simulink model "Sphere_Complex_Model"  (R2023a)
settings: Solver=VariableStepAuto  StartTime=0.0  StopTime=100  FixedStep=impulse_time  RelTol=1e-3
values from neighbouring files (symbols this model uses):
  Ex_Force = Command_Force(Input_F, F_Coord)    [init.m]    (also in nongrad_opt.m; obj_func.m; obj_func_plot.m)
  impulse_time = 0.001    [init.m]    (also in nongrad_opt.m; obj_func.m; obj_func_plot.m)
  Param = Sphere_Parameters(percent_foam, percent_metal)    [init.m]    (also in nongrad_opt.m = Sphere_Parameters(percent_foam(row), percent_metal(column)); obj_func.m; obj_func_plot.m = Sphere_Parameters(pf(row, column), pm(row, column)))
undefined symbols (not defined in the file or in its folder): Sphere_Model
settings Model: Creator=goks  LastModifiedBy=goks

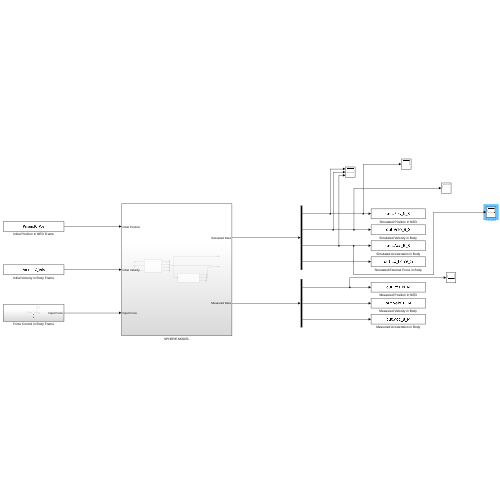
[thumbnail: Simulink's stored preview of the top-level diagram]
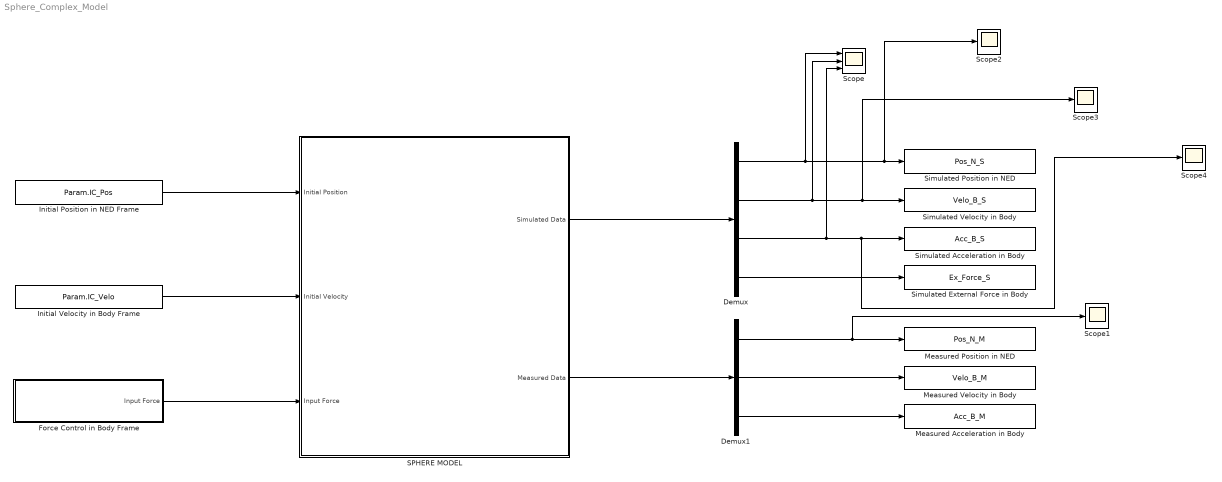
== system Sphere_Complex_Model ==
  Demux : Demux
  Demux1 : Demux  Outputs=3
  Force Control in Body Frame : Subsystem
  Initial Position in NED Frame : Constant  Value=Param.IC_Pos
  Initial Velocity in Body Frame : Constant  Value=Param.IC_Velo
  Measured Acceleration in Body : ToWorkspace  VariableName=Acc_B_M  SaveFormat=Timeseries  SampleTime=-1
  Measured Position in NED : ToWorkspace  VariableName=Pos_N_M  SaveFormat=Timeseries  SampleTime=-1
  Measured Velocity in Body : ToWorkspace  VariableName=Velo_B_M  SaveFormat=Timeseries  SampleTime=-1
  SPHERE MODEL : Subsystem
  Scope : Scope  NumInputPorts=3
  Scope{1..4} (4 alike) : Scope
  Simulated Acceleration in Body : ToWorkspace  VariableName=Acc_B_S  SaveFormat=Timeseries  SampleTime=-1
  Simulated External Force in Body : ToWorkspace  VariableName=Ex_Force_S  SaveFormat=Timeseries  SampleTime=-1
  Simulated Position in NED : ToWorkspace  VariableName=Pos_N_S  SaveFormat=Timeseries  SampleTime=-1
  Simulated Velocity in Body : ToWorkspace  VariableName=Velo_B_S  SaveFormat=Timeseries  SampleTime=-1
  wires:
  SPHERE MODEL/1(Simulated Data) -> Demux/1
  SPHERE MODEL/2(Measured Data) -> Demux1/1
  Demux/1 -> Scope/1, Scope2/1, Simulated Position in NED/1
  Demux/2 -> Scope/2, Scope3/1, Simulated Velocity in Body/1
  Demux/3 -> Scope/3, Scope4/1, Simulated Acceleration in Body/1
  Demux/4 -> Simulated External Force in Body/1
  Demux1/2 -> Measured Velocity in Body/1
  Demux1/3 -> Measured Acceleration in Body/1
  Initial Position in NED Frame/1 -> SPHERE MODEL/1("Initial Position ")
  Initial Velocity in Body Frame/1 -> SPHERE MODEL/2(Initial Velocity)
  Force Control in Body Frame/1(Input Force) -> SPHERE MODEL/3(Input Force)
  Demux1/1 -> Scope1/1, Measured Position in NED/1

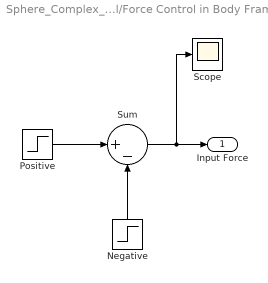
== system Sphere_Complex_Model/Force Control in Body Frame ==
  Negative : Step  Time=1+impulse_time  Before=zeros(6,1)  After=Ex_Force  SampleTime=0
  Positive : Step  Before=zeros(6,1)  After=Ex_Force  SampleTime=0
  Scope : Scope
  Sum : Sum  Inputs=|+-
  Input Force : Outport
  wires:
  Positive/1 -> Sum/1
  Negative/1 -> Sum/2
  Sum/1 -> Scope/1, Input Force/1

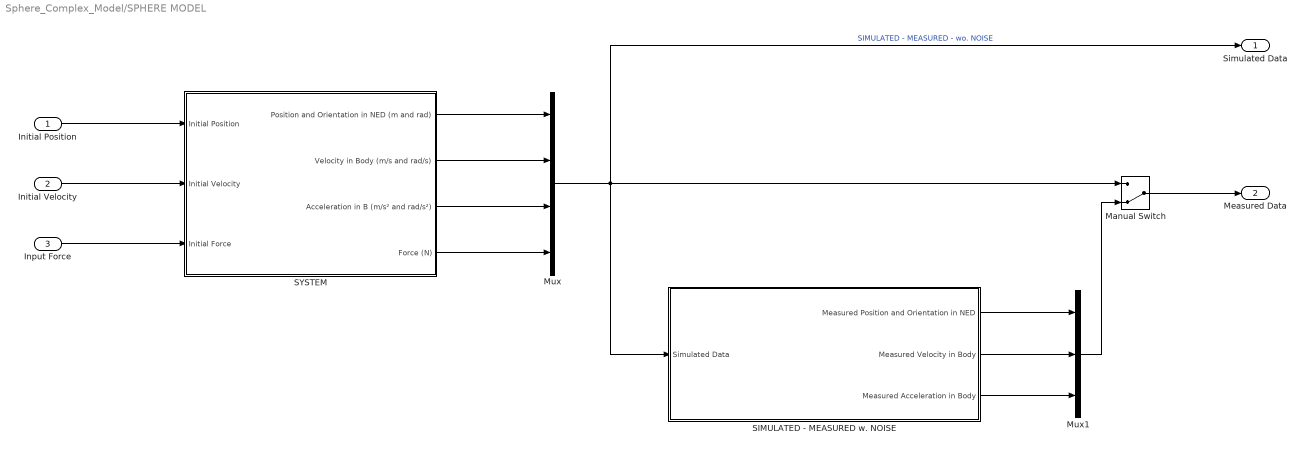
== system Sphere_Complex_Model/SPHERE MODEL ==
  "Initial Position " : Inport
  Initial Velocity : Inport  Port=2
  Input Force : Inport  Port=3
  Manual Switch : ManualSwitch  CurrentSetting=0
  Mux : Mux
  Mux1 : Mux  Inputs=3
  SIMULATED - MEASURED w. NOISE : Subsystem
  SYSTEM : Subsystem
  Simulated Data : Outport
  Measured Data : Outport  Port=2
  wires:
  SYSTEM/1(Position and Orientation in NED (m and rad)) -> Mux/1
  SYSTEM/2(Velocity in Body (m/s and rad/s)) -> Mux/2
  SYSTEM/3(Acceleration in B (m/s² and rad/s²)) -> Mux/3
  SYSTEM/4(Force (N)) -> Mux/4
  "Initial Position "/1 -> SYSTEM/1("Initial Position ")
  Initial Velocity/1 -> SYSTEM/2(Initial Velocity)
  Input Force/1 -> SYSTEM/3(Initial Force)
  SIMULATED - MEASURED w. NOISE/2(Measured Velocity in Body) -> Mux1/2
  SIMULATED - MEASURED w. NOISE/1(Measured Position and Orientation in NED) -> Mux1/1
  SIMULATED - MEASURED w. NOISE/3(Measured Acceleration in Body) -> Mux1/3
  Mux/1 -> SIMULATED - MEASURED w. NOISE/1(Simulated Data), Manual Switch/1, Simulated Data/1  "SIMULATED - MEASURED - wo. NOISE"
  Manual Switch/1 -> Measured Data/1
  Mux1/1 -> Manual Switch/2

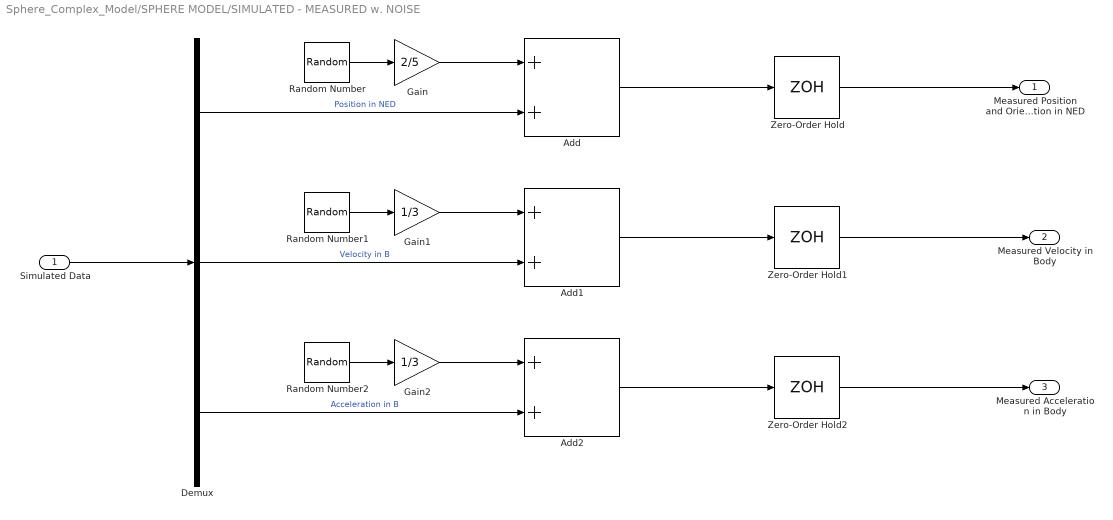
== system Sphere_Complex_Model/SPHERE MODEL/SIMULATED - MEASURED w. NOISE ==
  Simulated Data : Inport
  Add : Sum
  Add1 : Sum
  Add2 : Sum
  Demux : Demux  Outputs=3
  Gain : Gain  Gain=2/5
  Gain1 : Gain  Gain=1/3
  Gain2 : Gain  Gain=1/3
  Random Number : RandomNumber  Variance=0.01  SampleTime=0.01
  Random Number1 : RandomNumber  Variance=0.01  SampleTime=0.01
  Random Number2 : RandomNumber  Variance=0.01  SampleTime=0.01
  Zero-Order Hold : ZeroOrderHold  SampleTime=-1
  Zero-Order Hold1 : ZeroOrderHold  SampleTime=-1
  Zero-Order Hold2 : ZeroOrderHold  SampleTime=-1
  Measured Position and Orientation in NED : Outport
  Measured Velocity in Body : Outport  Port=2
  Measured Acceleration in Body : Outport  Port=3
  wires:
  Simulated Data/1 -> Demux/1
  Demux/1 -> Add/2  "Position in NED"
  Random Number/1 -> Gain/1
  Gain/1 -> Add/1
  Random Number1/1 -> Gain1/1
  Demux/2 -> Add1/2  "Velocity in B"
  Gain1/1 -> Add1/1
  Random Number2/1 -> Gain2/1
  Demux/3 -> Add2/2  "Acceleration in B"
  Gain2/1 -> Add2/1
  Add/1 -> Zero-Order Hold/1
  Add1/1 -> Zero-Order Hold1/1
  Add2/1 -> Zero-Order Hold2/1
  Zero-Order Hold/1 -> Measured Position and Orientation in NED/1
  Zero-Order Hold1/1 -> Measured Velocity in Body/1
  Zero-Order Hold2/1 -> Measured Acceleration in Body/1

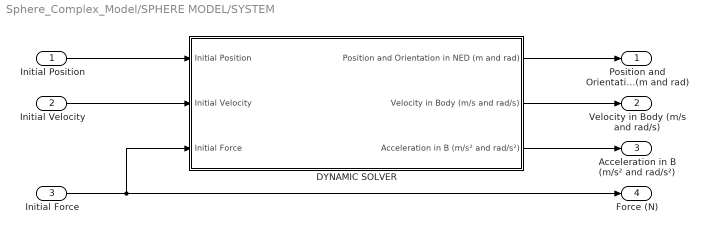
== system Sphere_Complex_Model/SPHERE MODEL/SYSTEM ==
  "Initial Position " : Inport
  Initial Velocity : Inport  Port=2
  Initial Force : Inport  Port=3
  DYNAMIC SOLVER : Subsystem
  Position and Orientation in NED (m and rad) : Outport
  Velocity in Body (m/s and rad/s) : Outport  Port=2
  Acceleration in B (m/s² and rad/s²) : Outport  Port=3
  Force (N) : Outport  Port=4
  wires:
  Initial Velocity/1 -> DYNAMIC SOLVER/2(Initial Velocity)
  "Initial Position "/1 -> DYNAMIC SOLVER/1("Initial Position ")
  DYNAMIC SOLVER/2(Velocity in Body (m/s and rad/s)) -> Velocity in Body (m/s and rad/s)/1
  DYNAMIC SOLVER/1(Position and Orientation in NED (m and rad)) -> Position and Orientation in NED (m and rad)/1
  DYNAMIC SOLVER/3(Acceleration in B (m/s² and rad/s²)) -> Acceleration in B (m/s² and rad/s²)/1
  Initial Force/1 -> Force (N)/1, DYNAMIC SOLVER/3(Initial Force)

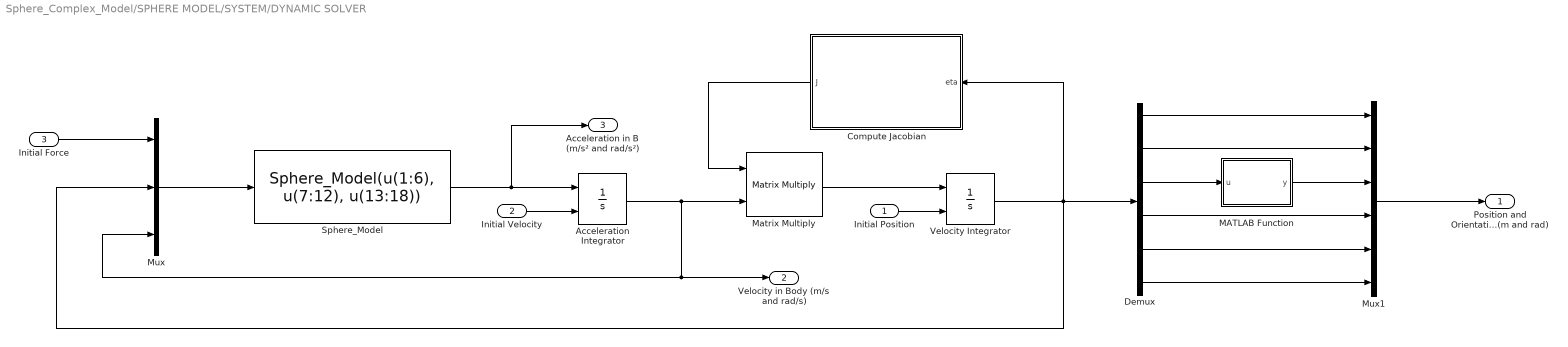
== system Sphere_Complex_Model/SPHERE MODEL/SYSTEM/DYNAMIC SOLVER ==
  "Initial Position " : Inport
  Initial Velocity : Inport  Port=2
  Initial Force : Inport  Port=3
  Acceleration Integrator : Integrator  InitialConditionSource=external
  Compute Jacobian : MATLAB Function  TreatAsAtomicUnit=on
  Demux : Demux  Outputs=6
  MATLAB Function : MATLAB Function  TreatAsAtomicUnit=on
  Matrix Multiply : Product  Multiplication=Matrix(*)
  Mux : Mux  Inputs=3
  Mux1 : Mux  Inputs=6
  "Sphere_Model " : MATLABFcn  MATLABFcn=Sphere_Model(u(1:6), u(7:12), u(13:18))  OutputDimensions=6
  Velocity Integrator : Integrator  InitialConditionSource=external
  Position and Orientation in NED (m and rad) : Outport
  Velocity in Body (m/s and rad/s) : Outport  Port=2
  Acceleration in B (m/s² and rad/s²) : Outport  Port=3
  wires:
  Mux/1 -> "Sphere_Model "/1
  "Sphere_Model "/1 -> Acceleration Integrator/1, Acceleration in B (m/s² and rad/s²)/1
  Initial Velocity/1 -> Acceleration Integrator/2
  Acceleration Integrator/1 -> Velocity in Body (m/s and rad/s)/1, Mux/3, Matrix Multiply/2
  Matrix Multiply/1 -> Velocity Integrator/1
  Initial Force/1 -> Mux/1
  "Initial Position "/1 -> Velocity Integrator/2
  Compute Jacobian/1(J) -> Matrix Multiply/1
  Velocity Integrator/1 -> Mux/2, Compute Jacobian/1(eta), Demux/1
  Demux/1 -> Mux1/1
  Demux/2 -> Mux1/2
  Demux/4 -> Mux1/4
  Demux/5 -> Mux1/5
  Demux/6 -> Mux1/6
  Demux/3 -> MATLAB Function/1(u)
  MATLAB Function/1(y) -> Mux1/3
  Mux1/1 -> Position and Orientation in NED (m and rad)/1

== matlab function Sphere_Complex_Model/SPHERE MODEL/SYSTEM/DYNAMIC SOLVER/Compute Jacobian ==
  data: eta input; J output
function J = Mapping(eta)

[~, ~, J] = Jacobian(eta);

end

== matlab function Sphere_Complex_Model/SPHERE MODEL/SYSTEM/DYNAMIC SOLVER/MATLAB Function ==
  data: u input; y output
function y = fcn(u)
if u > 0
    z = 0;
else
    z = u;
end
y = z;
